simulink model "controller_dev_sg_HIL_noTP"  (R2018b)
settings: configuration reference "Physics" (kept outside this file)
model workspace (MAT data in the model file):
  m = 1000
values from neighbouring files (symbols this model uses):
  bool_activate_Vehicles : value not decoded    [controller_dev_sg.sldd]
  ModObj_ObjList_SendPort = 11004.0    [UDPPortConfig.sldd]
  ModSens_GpsSenDat_SendPort = 3002.0    [UDPPortConfig.sldd]
  sensors_freq_camera = 37.0    [controller_dev_sg.sldd]
  sensors_freq_gps = 20.0    [controller_dev_sg.sldd]
  sensors_freq_imu = 100.0    [controller_dev_sg.sldd]
  sensors_freq_lidar = 12.0    [controller_dev_sg.sldd]
  sensors_freq_radar = 20.0    [controller_dev_sg.sldd]
undefined symbols (not defined in the file or in its folder): activate_VariableFriction, C, tpa_map_Reference, tSPhysics, x0_vehiclepos_start_veh1, x0_vehiclepos_start_veh10, x0_vehiclepos_start_veh2, x0_vehiclepos_start_veh3, x0_vehiclepos_start_veh4, x0_vehiclepos_start_veh5, x0_vehiclepos_start_veh6, x0_vehiclepos_start_veh7, x0_vehiclepos_start_veh8, x0_vehiclepos_start_veh9
libraries: xpcutilitieslib x273, xpcrtudplib x215, aerolibconvert2 x48, simulink x30, etargetslib x26, speedgoatlib_IO612 x7, canmsglib x6, slrtlib x4
(part 3 of 16)

== system controller_dev_sg_HIL_noTP/UDP to Control (Position, IMU, Wheelspeed)4 ==
  VehicleSensorData : Inport
  VehicleSystemStatus : Inport  Port=2
  ActuatorLimitations : Inport  Port=3
  Enable : EnablePort
  Bus Creator : BusCreator  Inputs=14
  Bus Creator2 : BusCreator  Inputs=4
  Bus Selector : BusSelector  OutputSignals=omega_WheelFL_radps,omega_WheelFR_radps,omega_WheelRL_radps,omega_WheelRR_radps,ax_CoGIMU1_mps2,ay_CoGIMU1_mps2,dPsi_YawRateIMU1_radps,Delta_Wheel_rad,p_BrakeF_bar,p_BrakeR_bar,ThrottlePos_perc,T_Engine_Nm,omega_Engine_radps,GearEngaged
  Bus Selector1 : BusSelector  OutputSignals=Hardware,AIDriver,ParkBrakeApplied_b,VehicleReady2Drive
  Bus Selector2 : BusSelector  OutputSignals=SteeringAngleMax_rad,SteeringAngleMin_rad,DriveForceMax_N,DriveForceMin_N
  Byte Packing 1 : xpcutilitieslib/Byte Packing   MaskPackedDataType=uint8  MaskUnpackedDataTypes={'uint16','uint16','uint8','uint8'}  MaskAlignment=1
  Byte Packing 2 : xpcutilitieslib/Byte Packing   MaskPackedDataType=uint8  MaskUnpackedDataTypes={'double'}  MaskAlignment=1
  Byte Packing 3 : xpcutilitieslib/Byte Packing   MaskPackedDataType=uint8  MaskUnpackedDataTypes={'double'}  MaskAlignment=1
  Data Type Conversion{,1..3,8..21} (18 alike) : DataTypeConversion  OutDataTypeStr=double
  Data Type Conversion4 : DataTypeConversion  OutDataTypeStr=uint16
  Data Type Conversion5 : DataTypeConversion  OutDataTypeStr=uint16
  Data Type Conversion6 : DataTypeConversion  OutDataTypeStr=uint8
  Data Type Conversion7 : DataTypeConversion  OutDataTypeStr=uint8
  UDP Send1 : xpcrtudplib/UDP Send  ipAddressVal=10.0.0.20  localPort=40550  toAddress=10.0.0.15  toPort=ModCtrl_VehSenDat_SendPort  sampleTime=-1
      settings: SourceProductName=Simulink Real-Time  SourceProductBaseCode=XP
  UDP Send2 : xpcrtudplib/UDP Send  ipAddressVal=10.0.0.20  localPort=40551  toAddress=10.0.0.15  toPort=ModCtrl_VehSysStat_SendPort  sampleTime=-1
      settings: SourceProductName=Simulink Real-Time  SourceProductBaseCode=XP
  UDP Send3 : xpcrtudplib/UDP Send  ipAddressVal=10.0.0.20  localPort=40552  toAddress=10.0.0.15  toPort=ModCtrl_ActLim_SendPort  sampleTime=-1
      settings: SourceProductName=Simulink Real-Time  SourceProductBaseCode=XP
  Width : Width
  Width1 : Width
  Width2 : Width
  wires:
  VehicleSensorData/1 -> Bus Selector/1
  Byte Packing 3/1 -> UDP Send1/1, Width/1
  Width/1 -> UDP Send1/2
  VehicleSystemStatus/1 -> Bus Selector1/1
  Bus Selector1/1 -> Data Type Conversion4/1  "<Hardware>"
  Bus Selector1/4 -> Data Type Conversion6/1  "<VehicleReady2Drive>"
  Bus Selector1/3 -> Data Type Conversion7/1  "<ParkBrakeApplied_b>"
  Bus Selector1/2 -> Data Type Conversion5/1  "<AIDriver>"
  ActuatorLimitations/1 -> Bus Selector2/1
  Bus Selector2/4 -> Data Type Conversion9/1  "<DriveForceMin_N>"
  Bus Selector2/3 -> Data Type Conversion10/1  "<DriveForceMax_N>"
  Bus Selector2/2 -> Data Type Conversion11/1  "<SteeringAngleMin_rad>"
  Bus Selector2/1 -> Data Type Conversion8/1  "<SteeringAngleMax_rad>"
  Data Type Conversion6/1 -> Byte Packing 1/4
  Data Type Conversion7/1 -> Byte Packing 1/3
  Data Type Conversion5/1 -> Byte Packing 1/2
  Data Type Conversion8/1 -> Bus Creator2/1
  Data Type Conversion11/1 -> Bus Creator2/2
  Data Type Conversion10/1 -> Bus Creator2/3
  Data Type Conversion9/1 -> Bus Creator2/4
  Bus Creator/1 -> Byte Packing 3/1
  Data Type Conversion4/1 -> Byte Packing 1/1
  Bus Creator2/1 -> Byte Packing 2/1
  Byte Packing 1/1 -> UDP Send2/1, Width1/1
  Width1/1 -> UDP Send2/2
  Byte Packing 2/1 -> UDP Send3/1, Width2/1
  Width2/1 -> UDP Send3/2
  Data Type Conversion1/1 -> Bus Creator/4
  Data Type Conversion2/1 -> Bus Creator/3
  Data Type Conversion19/1 -> Bus Creator/12
  Data Type Conversion3/1 -> Bus Creator/2
  Data Type Conversion16/1 -> Bus Creator/11
  Data Type Conversion14/1 -> Bus Creator/5
  Bus Selector/3 -> Data Type Conversion2/1  "<omega_WheelRL_radps>"
  Bus Selector/1 -> Data Type Conversion/1  "<omega_WheelFL_radps>"
  Data Type Conversion13/1 -> Bus Creator/7
  Bus Selector/4 -> Data Type Conversion1/1  "<omega_WheelRR_radps>"
  Bus Selector/2 -> Data Type Conversion3/1  "<omega_WheelFR_radps>"
  Data Type Conversion21/1 -> Bus Creator/9
  Data Type Conversion15/1 -> Bus Creator/8
  Bus Selector/10 -> Data Type Conversion20/1  "<p_BrakeR_bar>"
  Bus Selector/9 -> Data Type Conversion21/1  "<p_BrakeF_bar>"
  Bus Selector/8 -> Data Type Conversion15/1  "<Delta_Wheel_rad>"
  Data Type Conversion12/1 -> Bus Creator/6
  Data Type Conversion17/1 -> Bus Creator/13
  Bus Selector/12 -> Data Type Conversion19/1  "<T_Engine_Nm>"
  Bus Selector/13 -> Data Type Conversion17/1  "<omega_Engine_radps>"
  Bus Selector/11 -> Data Type Conversion16/1  "<ThrottlePos_perc>"
  Bus Selector/7 -> Data Type Conversion13/1  "<dPsi_YawRateIMU1_radps>"
  Data Type Conversion/1 -> Bus Creator/1
  Data Type Conversion20/1 -> Bus Creator/10
  Bus Selector/6 -> Data Type Conversion12/1  "<ay_CoGIMU1_mps2>"
  Data Type Conversion18/1 -> Bus Creator/14
  Bus Selector/5 -> Data Type Conversion14/1  "<ax_CoGIMU1_mps2>"
  Bus Selector/14 -> Data Type Conversion18/1  "<GearEngaged>"

== system controller_dev_sg_HIL_noTP/UDP to Control (Position, IMU, Wheelspeed)5 ==
  VehicleSensorData : Inport
  VehicleSystemStatus : Inport  Port=2
  ActuatorLimitations : Inport  Port=3
  Enable : EnablePort
  Bus Creator : BusCreator  Inputs=14
  Bus Creator2 : BusCreator  Inputs=4
  Bus Selector : BusSelector  OutputSignals=omega_WheelFL_radps,omega_WheelFR_radps,omega_WheelRL_radps,omega_WheelRR_radps,ax_CoGIMU1_mps2,ay_CoGIMU1_mps2,dPsi_YawRateIMU1_radps,Delta_Wheel_rad,p_BrakeF_bar,p_BrakeR_bar,ThrottlePos_perc,T_Engine_Nm,omega_Engine_radps,GearEngaged
  Bus Selector1 : BusSelector  OutputSignals=Hardware,AIDriver,ParkBrakeApplied_b,VehicleReady2Drive
  Bus Selector2 : BusSelector  OutputSignals=SteeringAngleMax_rad,SteeringAngleMin_rad,DriveForceMax_N,DriveForceMin_N
  Byte Packing 1 : xpcutilitieslib/Byte Packing   MaskPackedDataType=uint8  MaskUnpackedDataTypes={'uint16','uint16','uint8','uint8'}  MaskAlignment=1
  Byte Packing 2 : xpcutilitieslib/Byte Packing   MaskPackedDataType=uint8  MaskUnpackedDataTypes={'double'}  MaskAlignment=1
  Byte Packing 3 : xpcutilitieslib/Byte Packing   MaskPackedDataType=uint8  MaskUnpackedDataTypes={'double'}  MaskAlignment=1
  Data Type Conversion{,1..3,8..21} (18 alike) : DataTypeConversion  OutDataTypeStr=double
  Data Type Conversion4 : DataTypeConversion  OutDataTypeStr=uint16
  Data Type Conversion5 : DataTypeConversion  OutDataTypeStr=uint16
  Data Type Conversion6 : DataTypeConversion  OutDataTypeStr=uint8
  Data Type Conversion7 : DataTypeConversion  OutDataTypeStr=uint8
  UDP Send1 : xpcrtudplib/UDP Send  ipAddressVal=10.0.0.20  localPort=40560  toAddress=10.0.0.16  toPort=ModCtrl_VehSenDat_SendPort  sampleTime=-1
      settings: SourceProductName=Simulink Real-Time  SourceProductBaseCode=XP
  UDP Send2 : xpcrtudplib/UDP Send  ipAddressVal=10.0.0.20  localPort=40561  toAddress=10.0.0.16  toPort=ModCtrl_VehSysStat_SendPort  sampleTime=-1
      settings: SourceProductName=Simulink Real-Time  SourceProductBaseCode=XP
  UDP Send3 : xpcrtudplib/UDP Send  ipAddressVal=10.0.0.20  localPort=40562  toAddress=10.0.0.16  toPort=ModCtrl_ActLim_SendPort  sampleTime=-1
      settings: SourceProductName=Simulink Real-Time  SourceProductBaseCode=XP
  Width : Width
  Width1 : Width
  Width2 : Width
  wires:
  VehicleSensorData/1 -> Bus Selector/1
  Byte Packing 3/1 -> UDP Send1/1, Width/1
  Width/1 -> UDP Send1/2
  VehicleSystemStatus/1 -> Bus Selector1/1
  Bus Selector1/1 -> Data Type Conversion4/1  "<Hardware>"
  Bus Selector1/4 -> Data Type Conversion6/1  "<VehicleReady2Drive>"
  Bus Selector1/3 -> Data Type Conversion7/1  "<ParkBrakeApplied_b>"
  Bus Selector1/2 -> Data Type Conversion5/1  "<AIDriver>"
  ActuatorLimitations/1 -> Bus Selector2/1
  Bus Selector2/4 -> Data Type Conversion9/1  "<DriveForceMin_N>"
  Bus Selector2/3 -> Data Type Conversion10/1  "<DriveForceMax_N>"
  Bus Selector2/2 -> Data Type Conversion11/1  "<SteeringAngleMin_rad>"
  Bus Selector2/1 -> Data Type Conversion8/1  "<SteeringAngleMax_rad>"
  Data Type Conversion6/1 -> Byte Packing 1/4
  Data Type Conversion7/1 -> Byte Packing 1/3
  Data Type Conversion5/1 -> Byte Packing 1/2
  Data Type Conversion8/1 -> Bus Creator2/1
  Data Type Conversion11/1 -> Bus Creator2/2
  Data Type Conversion10/1 -> Bus Creator2/3
  Data Type Conversion9/1 -> Bus Creator2/4
  Bus Creator/1 -> Byte Packing 3/1
  Data Type Conversion4/1 -> Byte Packing 1/1
  Bus Creator2/1 -> Byte Packing 2/1
  Byte Packing 1/1 -> UDP Send2/1, Width1/1
  Width1/1 -> UDP Send2/2
  Byte Packing 2/1 -> UDP Send3/1, Width2/1
  Width2/1 -> UDP Send3/2
  Data Type Conversion1/1 -> Bus Creator/4
  Data Type Conversion2/1 -> Bus Creator/3
  Data Type Conversion19/1 -> Bus Creator/12
  Data Type Conversion3/1 -> Bus Creator/2
  Data Type Conversion16/1 -> Bus Creator/11
  Data Type Conversion14/1 -> Bus Creator/5
  Bus Selector/3 -> Data Type Conversion2/1  "<omega_WheelRL_radps>"
  Bus Selector/1 -> Data Type Conversion/1  "<omega_WheelFL_radps>"
  Data Type Conversion13/1 -> Bus Creator/7
  Bus Selector/4 -> Data Type Conversion1/1  "<omega_WheelRR_radps>"
  Bus Selector/2 -> Data Type Conversion3/1  "<omega_WheelFR_radps>"
  Data Type Conversion21/1 -> Bus Creator/9
  Data Type Conversion15/1 -> Bus Creator/8
  Bus Selector/10 -> Data Type Conversion20/1  "<p_BrakeR_bar>"
  Bus Selector/9 -> Data Type Conversion21/1  "<p_BrakeF_bar>"
  Bus Selector/8 -> Data Type Conversion15/1  "<Delta_Wheel_rad>"
  Data Type Conversion12/1 -> Bus Creator/6
  Data Type Conversion17/1 -> Bus Creator/13
  Bus Selector/12 -> Data Type Conversion19/1  "<T_Engine_Nm>"
  Bus Selector/13 -> Data Type Conversion17/1  "<omega_Engine_radps>"
  Bus Selector/11 -> Data Type Conversion16/1  "<ThrottlePos_perc>"
  Bus Selector/7 -> Data Type Conversion13/1  "<dPsi_YawRateIMU1_radps>"
  Data Type Conversion/1 -> Bus Creator/1
  Data Type Conversion20/1 -> Bus Creator/10
  Bus Selector/6 -> Data Type Conversion12/1  "<ay_CoGIMU1_mps2>"
  Data Type Conversion18/1 -> Bus Creator/14
  Bus Selector/5 -> Data Type Conversion14/1  "<ax_CoGIMU1_mps2>"
  Bus Selector/14 -> Data Type Conversion18/1  "<GearEngaged>"

== system controller_dev_sg_HIL_noTP/UDP to Control (Position, IMU, Wheelspeed)6 ==
  VehicleSensorData : Inport
  VehicleSystemStatus : Inport  Port=2
  ActuatorLimitations : Inport  Port=3
  Enable : EnablePort
  Bus Creator : BusCreator  Inputs=14
  Bus Creator2 : BusCreator  Inputs=4
  Bus Selector : BusSelector  OutputSignals=omega_WheelFL_radps,omega_WheelFR_radps,omega_WheelRL_radps,omega_WheelRR_radps,ax_CoGIMU1_mps2,ay_CoGIMU1_mps2,dPsi_YawRateIMU1_radps,Delta_Wheel_rad,p_BrakeF_bar,p_BrakeR_bar,ThrottlePos_perc,T_Engine_Nm,omega_Engine_radps,GearEngaged
  Bus Selector1 : BusSelector  OutputSignals=Hardware,AIDriver,ParkBrakeApplied_b,VehicleReady2Drive
  Bus Selector2 : BusSelector  OutputSignals=SteeringAngleMax_rad,SteeringAngleMin_rad,DriveForceMax_N,DriveForceMin_N
  Byte Packing 1 : xpcutilitieslib/Byte Packing   MaskPackedDataType=uint8  MaskUnpackedDataTypes={'uint16','uint16','uint8','uint8'}  MaskAlignment=1
  Byte Packing 2 : xpcutilitieslib/Byte Packing   MaskPackedDataType=uint8  MaskUnpackedDataTypes={'double'}  MaskAlignment=1
  Byte Packing 3 : xpcutilitieslib/Byte Packing   MaskPackedDataType=uint8  MaskUnpackedDataTypes={'double'}  MaskAlignment=1
  Data Type Conversion{,1..3,8..21} (18 alike) : DataTypeConversion  OutDataTypeStr=double
  Data Type Conversion4 : DataTypeConversion  OutDataTypeStr=uint16
  Data Type Conversion5 : DataTypeConversion  OutDataTypeStr=uint16
  Data Type Conversion6 : DataTypeConversion  OutDataTypeStr=uint8
  Data Type Conversion7 : DataTypeConversion  OutDataTypeStr=uint8
  UDP Send1 : xpcrtudplib/UDP Send  ipAddressVal=10.0.0.20  localPort=40570  toAddress=10.0.0.17  toPort=ModCtrl_VehSenDat_SendPort  sampleTime=-1
      settings: SourceProductName=Simulink Real-Time  SourceProductBaseCode=XP
  UDP Send2 : xpcrtudplib/UDP Send  ipAddressVal=10.0.0.20  localPort=40571  toAddress=10.0.0.17  toPort=ModCtrl_VehSysStat_SendPort  sampleTime=-1
      settings: SourceProductName=Simulink Real-Time  SourceProductBaseCode=XP
  UDP Send3 : xpcrtudplib/UDP Send  ipAddressVal=10.0.0.20  localPort=40572  toAddress=10.0.0.17  toPort=ModCtrl_ActLim_SendPort  sampleTime=-1
      settings: SourceProductName=Simulink Real-Time  SourceProductBaseCode=XP
  Width : Width
  Width1 : Width
  Width2 : Width
  wires:
  VehicleSensorData/1 -> Bus Selector/1
  Byte Packing 3/1 -> UDP Send1/1, Width/1
  Width/1 -> UDP Send1/2
  VehicleSystemStatus/1 -> Bus Selector1/1
  Bus Selector1/1 -> Data Type Conversion4/1  "<Hardware>"
  Bus Selector1/4 -> Data Type Conversion6/1  "<VehicleReady2Drive>"
  Bus Selector1/3 -> Data Type Conversion7/1  "<ParkBrakeApplied_b>"
  Bus Selector1/2 -> Data Type Conversion5/1  "<AIDriver>"
  ActuatorLimitations/1 -> Bus Selector2/1
  Bus Selector2/4 -> Data Type Conversion9/1  "<DriveForceMin_N>"
  Bus Selector2/3 -> Data Type Conversion10/1  "<DriveForceMax_N>"
  Bus Selector2/2 -> Data Type Conversion11/1  "<SteeringAngleMin_rad>"
  Bus Selector2/1 -> Data Type Conversion8/1  "<SteeringAngleMax_rad>"
  Data Type Conversion6/1 -> Byte Packing 1/4
  Data Type Conversion7/1 -> Byte Packing 1/3
  Data Type Conversion5/1 -> Byte Packing 1/2
  Data Type Conversion8/1 -> Bus Creator2/1
  Data Type Conversion11/1 -> Bus Creator2/2
  Data Type Conversion10/1 -> Bus Creator2/3
  Data Type Conversion9/1 -> Bus Creator2/4
  Bus Creator/1 -> Byte Packing 3/1
  Data Type Conversion4/1 -> Byte Packing 1/1
  Bus Creator2/1 -> Byte Packing 2/1
  Byte Packing 1/1 -> UDP Send2/1, Width1/1
  Width1/1 -> UDP Send2/2
  Byte Packing 2/1 -> UDP Send3/1, Width2/1
  Width2/1 -> UDP Send3/2
  Data Type Conversion1/1 -> Bus Creator/4
  Data Type Conversion2/1 -> Bus Creator/3
  Data Type Conversion19/1 -> Bus Creator/12
  Data Type Conversion3/1 -> Bus Creator/2
  Data Type Conversion16/1 -> Bus Creator/11
  Data Type Conversion14/1 -> Bus Creator/5
  Bus Selector/3 -> Data Type Conversion2/1  "<omega_WheelRL_radps>"
  Bus Selector/1 -> Data Type Conversion/1  "<omega_WheelFL_radps>"
  Data Type Conversion13/1 -> Bus Creator/7
  Bus Selector/4 -> Data Type Conversion1/1  "<omega_WheelRR_radps>"
  Bus Selector/2 -> Data Type Conversion3/1  "<omega_WheelFR_radps>"
  Data Type Conversion21/1 -> Bus Creator/9
  Data Type Conversion15/1 -> Bus Creator/8
  Bus Selector/10 -> Data Type Conversion20/1  "<p_BrakeR_bar>"
  Bus Selector/9 -> Data Type Conversion21/1  "<p_BrakeF_bar>"
  Bus Selector/8 -> Data Type Conversion15/1  "<Delta_Wheel_rad>"
  Data Type Conversion12/1 -> Bus Creator/6
  Data Type Conversion17/1 -> Bus Creator/13
  Bus Selector/12 -> Data Type Conversion19/1  "<T_Engine_Nm>"
  Bus Selector/13 -> Data Type Conversion17/1  "<omega_Engine_radps>"
  Bus Selector/11 -> Data Type Conversion16/1  "<ThrottlePos_perc>"
  Bus Selector/7 -> Data Type Conversion13/1  "<dPsi_YawRateIMU1_radps>"
  Data Type Conversion/1 -> Bus Creator/1
  Data Type Conversion20/1 -> Bus Creator/10
  Bus Selector/6 -> Data Type Conversion12/1  "<ay_CoGIMU1_mps2>"
  Data Type Conversion18/1 -> Bus Creator/14
  Bus Selector/5 -> Data Type Conversion14/1  "<ax_CoGIMU1_mps2>"
  Bus Selector/14 -> Data Type Conversion18/1  "<GearEngaged>"

== system controller_dev_sg_HIL_noTP/UDP to Control (Position, IMU, Wheelspeed)7 ==
  VehicleSensorData : Inport
  VehicleSystemStatus : Inport  Port=2
  ActuatorLimitations : Inport  Port=3
  Enable : EnablePort
  Bus Creator : BusCreator  Inputs=14
  Bus Creator2 : BusCreator  Inputs=4
  Bus Selector : BusSelector  OutputSignals=omega_WheelFL_radps,omega_WheelFR_radps,omega_WheelRL_radps,omega_WheelRR_radps,ax_CoGIMU1_mps2,ay_CoGIMU1_mps2,dPsi_YawRateIMU1_radps,Delta_Wheel_rad,p_BrakeF_bar,p_BrakeR_bar,ThrottlePos_perc,T_Engine_Nm,omega_Engine_radps,GearEngaged
  Bus Selector1 : BusSelector  OutputSignals=Hardware,AIDriver,ParkBrakeApplied_b,VehicleReady2Drive
  Bus Selector2 : BusSelector  OutputSignals=SteeringAngleMax_rad,SteeringAngleMin_rad,DriveForceMax_N,DriveForceMin_N
  Byte Packing 1 : xpcutilitieslib/Byte Packing   MaskPackedDataType=uint8  MaskUnpackedDataTypes={'uint16','uint16','uint8','uint8'}  MaskAlignment=1
  Byte Packing 2 : xpcutilitieslib/Byte Packing   MaskPackedDataType=uint8  MaskUnpackedDataTypes={'double'}  MaskAlignment=1
  Byte Packing 3 : xpcutilitieslib/Byte Packing   MaskPackedDataType=uint8  MaskUnpackedDataTypes={'double'}  MaskAlignment=1
  Data Type Conversion{,1..3,8..21} (18 alike) : DataTypeConversion  OutDataTypeStr=double
  Data Type Conversion4 : DataTypeConversion  OutDataTypeStr=uint16
  Data Type Conversion5 : DataTypeConversion  OutDataTypeStr=uint16
  Data Type Conversion6 : DataTypeConversion  OutDataTypeStr=uint8
  Data Type Conversion7 : DataTypeConversion  OutDataTypeStr=uint8
  UDP Send1 : xpcrtudplib/UDP Send  ipAddressVal=10.0.0.20  localPort=40580  toAddress=10.0.0.18  toPort=ModCtrl_VehSenDat_SendPort  sampleTime=-1
      settings: SourceProductName=Simulink Real-Time  SourceProductBaseCode=XP
  UDP Send2 : xpcrtudplib/UDP Send  ipAddressVal=10.0.0.20  localPort=40581  toAddress=10.0.0.18  toPort=ModCtrl_VehSysStat_SendPort  sampleTime=-1
      settings: SourceProductName=Simulink Real-Time  SourceProductBaseCode=XP
  UDP Send3 : xpcrtudplib/UDP Send  ipAddressVal=10.0.0.20  localPort=40582  toAddress=10.0.0.18  toPort=ModCtrl_ActLim_SendPort  sampleTime=-1
      settings: SourceProductName=Simulink Real-Time  SourceProductBaseCode=XP
  Width : Width
  Width1 : Width
  Width2 : Width
  wires:
  VehicleSensorData/1 -> Bus Selector/1
  Byte Packing 3/1 -> UDP Send1/1, Width/1
  Width/1 -> UDP Send1/2
  VehicleSystemStatus/1 -> Bus Selector1/1
  Bus Selector1/1 -> Data Type Conversion4/1  "<Hardware>"
  Bus Selector1/4 -> Data Type Conversion6/1  "<VehicleReady2Drive>"
  Bus Selector1/3 -> Data Type Conversion7/1  "<ParkBrakeApplied_b>"
  Bus Selector1/2 -> Data Type Conversion5/1  "<AIDriver>"
  ActuatorLimitations/1 -> Bus Selector2/1
  Bus Selector2/4 -> Data Type Conversion9/1  "<DriveForceMin_N>"
  Bus Selector2/3 -> Data Type Conversion10/1  "<DriveForceMax_N>"
  Bus Selector2/2 -> Data Type Conversion11/1  "<SteeringAngleMin_rad>"
  Bus Selector2/1 -> Data Type Conversion8/1  "<SteeringAngleMax_rad>"
  Data Type Conversion6/1 -> Byte Packing 1/4
  Data Type Conversion7/1 -> Byte Packing 1/3
  Data Type Conversion5/1 -> Byte Packing 1/2
  Data Type Conversion8/1 -> Bus Creator2/1
  Data Type Conversion11/1 -> Bus Creator2/2
  Data Type Conversion10/1 -> Bus Creator2/3
  Data Type Conversion9/1 -> Bus Creator2/4
  Bus Creator/1 -> Byte Packing 3/1
  Data Type Conversion4/1 -> Byte Packing 1/1
  Bus Creator2/1 -> Byte Packing 2/1
  Byte Packing 1/1 -> UDP Send2/1, Width1/1
  Width1/1 -> UDP Send2/2
  Byte Packing 2/1 -> UDP Send3/1, Width2/1
  Width2/1 -> UDP Send3/2
  Data Type Conversion1/1 -> Bus Creator/4
  Data Type Conversion2/1 -> Bus Creator/3
  Data Type Conversion19/1 -> Bus Creator/12
  Data Type Conversion3/1 -> Bus Creator/2
  Data Type Conversion16/1 -> Bus Creator/11
  Data Type Conversion14/1 -> Bus Creator/5
  Bus Selector/3 -> Data Type Conversion2/1  "<omega_WheelRL_radps>"
  Bus Selector/1 -> Data Type Conversion/1  "<omega_WheelFL_radps>"
  Data Type Conversion13/1 -> Bus Creator/7
  Bus Selector/4 -> Data Type Conversion1/1  "<omega_WheelRR_radps>"
  Bus Selector/2 -> Data Type Conversion3/1  "<omega_WheelFR_radps>"
  Data Type Conversion21/1 -> Bus Creator/9
  Data Type Conversion15/1 -> Bus Creator/8
  Bus Selector/10 -> Data Type Conversion20/1  "<p_BrakeR_bar>"
  Bus Selector/9 -> Data Type Conversion21/1  "<p_BrakeF_bar>"
  Bus Selector/8 -> Data Type Conversion15/1  "<Delta_Wheel_rad>"
  Data Type Conversion12/1 -> Bus Creator/6
  Data Type Conversion17/1 -> Bus Creator/13
  Bus Selector/12 -> Data Type Conversion19/1  "<T_Engine_Nm>"
  Bus Selector/13 -> Data Type Conversion17/1  "<omega_Engine_radps>"
  Bus Selector/11 -> Data Type Conversion16/1  "<ThrottlePos_perc>"
  Bus Selector/7 -> Data Type Conversion13/1  "<dPsi_YawRateIMU1_radps>"
  Data Type Conversion/1 -> Bus Creator/1
  Data Type Conversion20/1 -> Bus Creator/10
  Bus Selector/6 -> Data Type Conversion12/1  "<ay_CoGIMU1_mps2>"
  Data Type Conversion18/1 -> Bus Creator/14
  Bus Selector/5 -> Data Type Conversion14/1  "<ax_CoGIMU1_mps2>"
  Bus Selector/14 -> Data Type Conversion18/1  "<GearEngaged>"

== system controller_dev_sg_HIL_noTP/UDP to Mapping and Localization (Position, IMU, Wheelspeed) ==
  VehicleSensorData : Inport
  Enable : EnablePort
  Bus Creator : BusCreator  Inputs=12
  Bus Selector : BusSelector  OutputSignals=x_Loc1_m,y_Loc1_m,psi_YawAngleLoc1_rad,vx_CoGVel1_mps,vy_CoGVel1_mps,dPsi_YawRateIMU1_radps,ax_CoGIMU1_mps2,ay_CoGIMU1_mps2,omega_WheelFL_radps,omega_WheelFR_radps,omega_WheelRL_radps,omega_WheelRR_radps
  Byte Packing 3 : xpcutilitieslib/Byte Packing   MaskPackedDataType=uint8  MaskUnpackedDataTypes={'double'}  MaskAlignment=1
  Data Type Conversion{,1..8,12..14} (12 alike) : DataTypeConversion  OutDataTypeStr=double
  UDP Send1 : xpcrtudplib/UDP Send  ipAddressVal=10.0.0.20  localPort=40513  toAddress=10.0.0.11  toPort=ModMapLoc_VehSenDat_SendPort  sampleTime=-1
      settings: SourceProductName=Simulink Real-Time  SourceProductBaseCode=XP
  Width : Width
  wires:
  VehicleSensorData/1 -> Bus Selector/1
  Byte Packing 3/1 -> Width/1, UDP Send1/1
  Width/1 -> UDP Send1/2
  Bus Creator/1 -> Byte Packing 3/1
  Bus Selector/12 -> Data Type Conversion13/1  "<omega_WheelRR_radps>"
  Bus Selector/11 -> Data Type Conversion12/1  "<omega_WheelRL_radps>"
  Bus Selector/10 -> Data Type Conversion14/1  "<omega_WheelFR_radps>"
  Bus Selector/9 -> Data Type Conversion1/1  "<omega_WheelFL_radps>"
  Bus Selector/7 -> Data Type Conversion3/1  "<ax_CoGIMU1_mps2>"
  Bus Selector/8 -> Data Type Conversion2/1  "<ay_CoGIMU1_mps2>"
  Bus Selector/6 -> Data Type Conversion/1  "<dPsi_YawRateIMU1_radps>"
  Bus Selector/1 -> Data Type Conversion4/1  "<x_Loc1_m>"
  Bus Selector/2 -> Data Type Conversion8/1  "<y_Loc1_m>"
  Bus Selector/3 -> Data Type Conversion7/1  "<psi_YawAngleLoc1_rad>"
  Bus Selector/4 -> Data Type Conversion5/1  "<vx_CoGVel1_mps>"
  Bus Selector/5 -> Data Type Conversion6/1  "<vy_CoGVel1_mps>"
  Data Type Conversion12/1 -> Bus Creator/11
  Data Type Conversion13/1 -> Bus Creator/12
  Data Type Conversion14/1 -> Bus Creator/10
  Data Type Conversion1/1 -> Bus Creator/9
  Data Type Conversion3/1 -> Bus Creator/7
  Data Type Conversion2/1 -> Bus Creator/8
  Data Type Conversion/1 -> Bus Creator/6
  Data Type Conversion6/1 -> Bus Creator/5
  Data Type Conversion5/1 -> Bus Creator/4
  Data Type Conversion7/1 -> Bus Creator/3
  Data Type Conversion8/1 -> Bus Creator/2
  Data Type Conversion4/1 -> Bus Creator/1

== system controller_dev_sg_HIL_noTP/UDP to Mapping and Localization (Position, IMU, Wheelspeed)1 ==
  VehicleSensorData : Inport
  Enable : EnablePort
  Bus Creator : BusCreator  Inputs=12
  Bus Selector : BusSelector  OutputSignals=x_Loc1_m,y_Loc1_m,psi_YawAngleLoc1_rad,vx_CoGVel1_mps,vy_CoGVel1_mps,dPsi_YawRateIMU1_radps,ax_CoGIMU1_mps2,ay_CoGIMU1_mps2,omega_WheelFL_radps,omega_WheelFR_radps,omega_WheelRL_radps,omega_WheelRR_radps
  Byte Packing 3 : xpcutilitieslib/Byte Packing   MaskPackedDataType=uint8  MaskUnpackedDataTypes={'double'}  MaskAlignment=1
  Data Type Conversion{,1..8,12..14} (12 alike) : DataTypeConversion  OutDataTypeStr=double
  UDP Send1 : xpcrtudplib/UDP Send  ipAddressVal=10.0.0.20  localPort=40523  toAddress=10.0.0.12  toPort=ModMapLoc_VehSenDat_SendPort  sampleTime=-1
      settings: SourceProductName=Simulink Real-Time  SourceProductBaseCode=XP
  Width : Width
  wires:
  VehicleSensorData/1 -> Bus Selector/1
  Byte Packing 3/1 -> Width/1, UDP Send1/1
  Width/1 -> UDP Send1/2
  Bus Creator/1 -> Byte Packing 3/1
  Bus Selector/12 -> Data Type Conversion13/1  "<omega_WheelRR_radps>"
  Bus Selector/11 -> Data Type Conversion12/1  "<omega_WheelRL_radps>"
  Bus Selector/10 -> Data Type Conversion14/1  "<omega_WheelFR_radps>"
  Bus Selector/9 -> Data Type Conversion1/1  "<omega_WheelFL_radps>"
  Bus Selector/7 -> Data Type Conversion3/1  "<ax_CoGIMU1_mps2>"
  Bus Selector/8 -> Data Type Conversion2/1  "<ay_CoGIMU1_mps2>"
  Bus Selector/6 -> Data Type Conversion/1  "<dPsi_YawRateIMU1_radps>"
  Bus Selector/1 -> Data Type Conversion4/1  "<x_Loc1_m>"
  Bus Selector/2 -> Data Type Conversion8/1  "<y_Loc1_m>"
  Bus Selector/3 -> Data Type Conversion7/1  "<psi_YawAngleLoc1_rad>"
  Bus Selector/4 -> Data Type Conversion5/1  "<vx_CoGVel1_mps>"
  Bus Selector/5 -> Data Type Conversion6/1  "<vy_CoGVel1_mps>"
  Data Type Conversion12/1 -> Bus Creator/11
  Data Type Conversion13/1 -> Bus Creator/12
  Data Type Conversion14/1 -> Bus Creator/10
  Data Type Conversion1/1 -> Bus Creator/9
  Data Type Conversion3/1 -> Bus Creator/7
  Data Type Conversion2/1 -> Bus Creator/8
  Data Type Conversion/1 -> Bus Creator/6
  Data Type Conversion6/1 -> Bus Creator/5
  Data Type Conversion5/1 -> Bus Creator/4
  Data Type Conversion7/1 -> Bus Creator/3
  Data Type Conversion8/1 -> Bus Creator/2
  Data Type Conversion4/1 -> Bus Creator/1

== system controller_dev_sg_HIL_noTP/UDP to Mapping and Localization (Position, IMU, Wheelspeed)2 ==
  VehicleSensorData : Inport
  Enable : EnablePort
  Bus Creator : BusCreator  Inputs=12
  Bus Selector : BusSelector  OutputSignals=x_Loc1_m,y_Loc1_m,psi_YawAngleLoc1_rad,vx_CoGVel1_mps,vy_CoGVel1_mps,dPsi_YawRateIMU1_radps,ax_CoGIMU1_mps2,ay_CoGIMU1_mps2,omega_WheelFL_radps,omega_WheelFR_radps,omega_WheelRL_radps,omega_WheelRR_radps
  Byte Packing 3 : xpcutilitieslib/Byte Packing   MaskPackedDataType=uint8  MaskUnpackedDataTypes={'double'}  MaskAlignment=1
  Data Type Conversion{,1..8,12..14} (12 alike) : DataTypeConversion  OutDataTypeStr=double
  UDP Send1 : xpcrtudplib/UDP Send  ipAddressVal=10.0.0.20  localPort=40533  toAddress=10.0.0.13  toPort=ModMapLoc_VehSenDat_SendPort  sampleTime=-1
      settings: SourceProductName=Simulink Real-Time  SourceProductBaseCode=XP
  Width : Width
  wires:
  VehicleSensorData/1 -> Bus Selector/1
  Byte Packing 3/1 -> Width/1, UDP Send1/1
  Width/1 -> UDP Send1/2
  Bus Creator/1 -> Byte Packing 3/1
  Bus Selector/12 -> Data Type Conversion13/1  "<omega_WheelRR_radps>"
  Bus Selector/11 -> Data Type Conversion12/1  "<omega_WheelRL_radps>"
  Bus Selector/10 -> Data Type Conversion14/1  "<omega_WheelFR_radps>"
  Bus Selector/9 -> Data Type Conversion1/1  "<omega_WheelFL_radps>"
  Bus Selector/7 -> Data Type Conversion3/1  "<ax_CoGIMU1_mps2>"
  Bus Selector/8 -> Data Type Conversion2/1  "<ay_CoGIMU1_mps2>"
  Bus Selector/6 -> Data Type Conversion/1  "<dPsi_YawRateIMU1_radps>"
  Bus Selector/1 -> Data Type Conversion4/1  "<x_Loc1_m>"
  Bus Selector/2 -> Data Type Conversion8/1  "<y_Loc1_m>"
  Bus Selector/3 -> Data Type Conversion7/1  "<psi_YawAngleLoc1_rad>"
  Bus Selector/4 -> Data Type Conversion5/1  "<vx_CoGVel1_mps>"
  Bus Selector/5 -> Data Type Conversion6/1  "<vy_CoGVel1_mps>"
  Data Type Conversion12/1 -> Bus Creator/11
  Data Type Conversion13/1 -> Bus Creator/12
  Data Type Conversion14/1 -> Bus Creator/10
  Data Type Conversion1/1 -> Bus Creator/9
  Data Type Conversion3/1 -> Bus Creator/7
  Data Type Conversion2/1 -> Bus Creator/8
  Data Type Conversion/1 -> Bus Creator/6
  Data Type Conversion6/1 -> Bus Creator/5
  Data Type Conversion5/1 -> Bus Creator/4
  Data Type Conversion7/1 -> Bus Creator/3
  Data Type Conversion8/1 -> Bus Creator/2
  Data Type Conversion4/1 -> Bus Creator/1

== system controller_dev_sg_HIL_noTP/UDP to Mapping and Localization (Position, IMU, Wheelspeed)3 ==
  VehicleSensorData : Inport
  Enable : EnablePort
  Bus Creator : BusCreator  Inputs=12
  Bus Selector : BusSelector  OutputSignals=x_Loc1_m,y_Loc1_m,psi_YawAngleLoc1_rad,vx_CoGVel1_mps,vy_CoGVel1_mps,dPsi_YawRateIMU1_radps,ax_CoGIMU1_mps2,ay_CoGIMU1_mps2,omega_WheelFL_radps,omega_WheelFR_radps,omega_WheelRL_radps,omega_WheelRR_radps
  Byte Packing 3 : xpcutilitieslib/Byte Packing   MaskPackedDataType=uint8  MaskUnpackedDataTypes={'double'}  MaskAlignment=1
  Data Type Conversion{,1..8,12..14} (12 alike) : DataTypeConversion  OutDataTypeStr=double
  UDP Send1 : xpcrtudplib/UDP Send  ipAddressVal=10.0.0.20  localPort=40543  toAddress=10.0.0.14  toPort=ModMapLoc_VehSenDat_SendPort  sampleTime=-1
      settings: SourceProductName=Simulink Real-Time  SourceProductBaseCode=XP
  Width : Width
  wires:
  VehicleSensorData/1 -> Bus Selector/1
  Byte Packing 3/1 -> Width/1, UDP Send1/1
  Width/1 -> UDP Send1/2
  Bus Creator/1 -> Byte Packing 3/1
  Bus Selector/12 -> Data Type Conversion13/1  "<omega_WheelRR_radps>"
  Bus Selector/11 -> Data Type Conversion12/1  "<omega_WheelRL_radps>"
  Bus Selector/10 -> Data Type Conversion14/1  "<omega_WheelFR_radps>"
  Bus Selector/9 -> Data Type Conversion1/1  "<omega_WheelFL_radps>"
  Bus Selector/7 -> Data Type Conversion3/1  "<ax_CoGIMU1_mps2>"
  Bus Selector/8 -> Data Type Conversion2/1  "<ay_CoGIMU1_mps2>"
  Bus Selector/6 -> Data Type Conversion/1  "<dPsi_YawRateIMU1_radps>"
  Bus Selector/1 -> Data Type Conversion4/1  "<x_Loc1_m>"
  Bus Selector/2 -> Data Type Conversion8/1  "<y_Loc1_m>"
  Bus Selector/3 -> Data Type Conversion7/1  "<psi_YawAngleLoc1_rad>"
  Bus Selector/4 -> Data Type Conversion5/1  "<vx_CoGVel1_mps>"
  Bus Selector/5 -> Data Type Conversion6/1  "<vy_CoGVel1_mps>"
  Data Type Conversion12/1 -> Bus Creator/11
  Data Type Conversion13/1 -> Bus Creator/12
  Data Type Conversion14/1 -> Bus Creator/10
  Data Type Conversion1/1 -> Bus Creator/9
  Data Type Conversion3/1 -> Bus Creator/7
  Data Type Conversion2/1 -> Bus Creator/8
  Data Type Conversion/1 -> Bus Creator/6
  Data Type Conversion6/1 -> Bus Creator/5
  Data Type Conversion5/1 -> Bus Creator/4
  Data Type Conversion7/1 -> Bus Creator/3
  Data Type Conversion8/1 -> Bus Creator/2
  Data Type Conversion4/1 -> Bus Creator/1

== system controller_dev_sg_HIL_noTP/UDP to Mapping and Localization (Position, IMU, Wheelspeed)4 ==
  VehicleSensorData : Inport
  Enable : EnablePort
  Bus Creator : BusCreator  Inputs=12
  Bus Selector : BusSelector  OutputSignals=x_Loc1_m,y_Loc1_m,psi_YawAngleLoc1_rad,vx_CoGVel1_mps,vy_CoGVel1_mps,dPsi_YawRateIMU1_radps,ax_CoGIMU1_mps2,ay_CoGIMU1_mps2,omega_WheelFL_radps,omega_WheelFR_radps,omega_WheelRL_radps,omega_WheelRR_radps
  Byte Packing 3 : xpcutilitieslib/Byte Packing   MaskPackedDataType=uint8  MaskUnpackedDataTypes={'double'}  MaskAlignment=1
  Data Type Conversion{,1..8,12..14} (12 alike) : DataTypeConversion  OutDataTypeStr=double
  UDP Send1 : xpcrtudplib/UDP Send  ipAddressVal=10.0.0.20  localPort=40553  toAddress=10.0.0.15  toPort=ModMapLoc_VehSenDat_SendPort  sampleTime=-1
      settings: SourceProductName=Simulink Real-Time  SourceProductBaseCode=XP
  Width : Width
  wires:
  VehicleSensorData/1 -> Bus Selector/1
  Byte Packing 3/1 -> Width/1, UDP Send1/1
  Width/1 -> UDP Send1/2
  Bus Creator/1 -> Byte Packing 3/1
  Bus Selector/12 -> Data Type Conversion13/1  "<omega_WheelRR_radps>"
  Bus Selector/11 -> Data Type Conversion12/1  "<omega_WheelRL_radps>"
  Bus Selector/10 -> Data Type Conversion14/1  "<omega_WheelFR_radps>"
  Bus Selector/9 -> Data Type Conversion1/1  "<omega_WheelFL_radps>"
  Bus Selector/7 -> Data Type Conversion3/1  "<ax_CoGIMU1_mps2>"
  Bus Selector/8 -> Data Type Conversion2/1  "<ay_CoGIMU1_mps2>"
  Bus Selector/6 -> Data Type Conversion/1  "<dPsi_YawRateIMU1_radps>"
  Bus Selector/1 -> Data Type Conversion4/1  "<x_Loc1_m>"
  Bus Selector/2 -> Data Type Conversion8/1  "<y_Loc1_m>"
  Bus Selector/3 -> Data Type Conversion7/1  "<psi_YawAngleLoc1_rad>"
  Bus Selector/4 -> Data Type Conversion5/1  "<vx_CoGVel1_mps>"
  Bus Selector/5 -> Data Type Conversion6/1  "<vy_CoGVel1_mps>"
  Data Type Conversion12/1 -> Bus Creator/11
  Data Type Conversion13/1 -> Bus Creator/12
  Data Type Conversion14/1 -> Bus Creator/10
  Data Type Conversion1/1 -> Bus Creator/9
  Data Type Conversion3/1 -> Bus Creator/7
  Data Type Conversion2/1 -> Bus Creator/8
  Data Type Conversion/1 -> Bus Creator/6
  Data Type Conversion6/1 -> Bus Creator/5
  Data Type Conversion5/1 -> Bus Creator/4
  Data Type Conversion7/1 -> Bus Creator/3
  Data Type Conversion8/1 -> Bus Creator/2
  Data Type Conversion4/1 -> Bus Creator/1

== system controller_dev_sg_HIL_noTP/UDP to Mapping and Localization (Position, IMU, Wheelspeed)5 ==
  VehicleSensorData : Inport
  Enable : EnablePort
  Bus Creator : BusCreator  Inputs=12
  Bus Selector : BusSelector  OutputSignals=x_Loc1_m,y_Loc1_m,psi_YawAngleLoc1_rad,vx_CoGVel1_mps,vy_CoGVel1_mps,dPsi_YawRateIMU1_radps,ax_CoGIMU1_mps2,ay_CoGIMU1_mps2,omega_WheelFL_radps,omega_WheelFR_radps,omega_WheelRL_radps,omega_WheelRR_radps
  Byte Packing 3 : xpcutilitieslib/Byte Packing   MaskPackedDataType=uint8  MaskUnpackedDataTypes={'double'}  MaskAlignment=1
  Data Type Conversion{,1..8,12..14} (12 alike) : DataTypeConversion  OutDataTypeStr=double
  UDP Send1 : xpcrtudplib/UDP Send  ipAddressVal=10.0.0.20  localPort=40563  toAddress=10.0.0.16  toPort=ModMapLoc_VehSenDat_SendPort  sampleTime=-1
      settings: SourceProductName=Simulink Real-Time  SourceProductBaseCode=XP
  Width : Width
  wires:
  VehicleSensorData/1 -> Bus Selector/1
  Byte Packing 3/1 -> Width/1, UDP Send1/1
  Width/1 -> UDP Send1/2
  Bus Creator/1 -> Byte Packing 3/1
  Bus Selector/12 -> Data Type Conversion13/1  "<omega_WheelRR_radps>"
  Bus Selector/11 -> Data Type Conversion12/1  "<omega_WheelRL_radps>"
  Bus Selector/10 -> Data Type Conversion14/1  "<omega_WheelFR_radps>"
  Bus Selector/9 -> Data Type Conversion1/1  "<omega_WheelFL_radps>"
  Bus Selector/7 -> Data Type Conversion3/1  "<ax_CoGIMU1_mps2>"
  Bus Selector/8 -> Data Type Conversion2/1  "<ay_CoGIMU1_mps2>"
  Bus Selector/6 -> Data Type Conversion/1  "<dPsi_YawRateIMU1_radps>"
  Bus Selector/1 -> Data Type Conversion4/1  "<x_Loc1_m>"
  Bus Selector/2 -> Data Type Conversion8/1  "<y_Loc1_m>"
  Bus Selector/3 -> Data Type Conversion7/1  "<psi_YawAngleLoc1_rad>"
  Bus Selector/4 -> Data Type Conversion5/1  "<vx_CoGVel1_mps>"
  Bus Selector/5 -> Data Type Conversion6/1  "<vy_CoGVel1_mps>"
  Data Type Conversion12/1 -> Bus Creator/11
  Data Type Conversion13/1 -> Bus Creator/12
  Data Type Conversion14/1 -> Bus Creator/10
  Data Type Conversion1/1 -> Bus Creator/9
  Data Type Conversion3/1 -> Bus Creator/7
  Data Type Conversion2/1 -> Bus Creator/8
  Data Type Conversion/1 -> Bus Creator/6
  Data Type Conversion6/1 -> Bus Creator/5
  Data Type Conversion5/1 -> Bus Creator/4
  Data Type Conversion7/1 -> Bus Creator/3
  Data Type Conversion8/1 -> Bus Creator/2
  Data Type Conversion4/1 -> Bus Creator/1

== system controller_dev_sg_HIL_noTP/UDP to Mapping and Localization (Position, IMU, Wheelspeed)6 ==
  VehicleSensorData : Inport
  Enable : EnablePort
  Bus Creator : BusCreator  Inputs=12
  Bus Selector : BusSelector  OutputSignals=x_Loc1_m,y_Loc1_m,psi_YawAngleLoc1_rad,vx_CoGVel1_mps,vy_CoGVel1_mps,dPsi_YawRateIMU1_radps,ax_CoGIMU1_mps2,ay_CoGIMU1_mps2,omega_WheelFL_radps,omega_WheelFR_radps,omega_WheelRL_radps,omega_WheelRR_radps
  Byte Packing 3 : xpcutilitieslib/Byte Packing   MaskPackedDataType=uint8  MaskUnpackedDataTypes={'double'}  MaskAlignment=1
  Data Type Conversion{,1..8,12..14} (12 alike) : DataTypeConversion  OutDataTypeStr=double
  UDP Send1 : xpcrtudplib/UDP Send  ipAddressVal=10.0.0.20  localPort=40573  toAddress=10.0.0.17  toPort=ModMapLoc_VehSenDat_SendPort  sampleTime=-1
      settings: SourceProductName=Simulink Real-Time  SourceProductBaseCode=XP
  Width : Width
  wires:
  VehicleSensorData/1 -> Bus Selector/1
  Byte Packing 3/1 -> Width/1, UDP Send1/1
  Width/1 -> UDP Send1/2
  Bus Creator/1 -> Byte Packing 3/1
  Bus Selector/12 -> Data Type Conversion13/1  "<omega_WheelRR_radps>"
  Bus Selector/11 -> Data Type Conversion12/1  "<omega_WheelRL_radps>"
  Bus Selector/10 -> Data Type Conversion14/1  "<omega_WheelFR_radps>"
  Bus Selector/9 -> Data Type Conversion1/1  "<omega_WheelFL_radps>"
  Bus Selector/7 -> Data Type Conversion3/1  "<ax_CoGIMU1_mps2>"
  Bus Selector/8 -> Data Type Conversion2/1  "<ay_CoGIMU1_mps2>"
  Bus Selector/6 -> Data Type Conversion/1  "<dPsi_YawRateIMU1_radps>"
  Bus Selector/1 -> Data Type Conversion4/1  "<x_Loc1_m>"
  Bus Selector/2 -> Data Type Conversion8/1  "<y_Loc1_m>"
  Bus Selector/3 -> Data Type Conversion7/1  "<psi_YawAngleLoc1_rad>"
  Bus Selector/4 -> Data Type Conversion5/1  "<vx_CoGVel1_mps>"
  Bus Selector/5 -> Data Type Conversion6/1  "<vy_CoGVel1_mps>"
  Data Type Conversion12/1 -> Bus Creator/11
  Data Type Conversion13/1 -> Bus Creator/12
  Data Type Conversion14/1 -> Bus Creator/10
  Data Type Conversion1/1 -> Bus Creator/9
  Data Type Conversion3/1 -> Bus Creator/7
  Data Type Conversion2/1 -> Bus Creator/8
  Data Type Conversion/1 -> Bus Creator/6
  Data Type Conversion6/1 -> Bus Creator/5
  Data Type Conversion5/1 -> Bus Creator/4
  Data Type Conversion7/1 -> Bus Creator/3
  Data Type Conversion8/1 -> Bus Creator/2
  Data Type Conversion4/1 -> Bus Creator/1

== system controller_dev_sg_HIL_noTP/UDP to Mapping and Localization (Position, IMU, Wheelspeed)7 ==
  VehicleSensorData : Inport
  Enable : EnablePort
  Bus Creator : BusCreator  Inputs=12
  Bus Selector : BusSelector  OutputSignals=x_Loc1_m,y_Loc1_m,psi_YawAngleLoc1_rad,vx_CoGVel1_mps,vy_CoGVel1_mps,dPsi_YawRateIMU1_radps,ax_CoGIMU1_mps2,ay_CoGIMU1_mps2,omega_WheelFL_radps,omega_WheelFR_radps,omega_WheelRL_radps,omega_WheelRR_radps
  Byte Packing 3 : xpcutilitieslib/Byte Packing   MaskPackedDataType=uint8  MaskUnpackedDataTypes={'double'}  MaskAlignment=1
  Data Type Conversion{,1..8,12..14} (12 alike) : DataTypeConversion  OutDataTypeStr=double
  UDP Send1 : xpcrtudplib/UDP Send  ipAddressVal=10.0.0.20  localPort=40583  toAddress=10.0.0.18  toPort=ModMapLoc_VehSenDat_SendPort  sampleTime=-1
      settings: SourceProductName=Simulink Real-Time  SourceProductBaseCode=XP
  Width : Width
  wires:
  VehicleSensorData/1 -> Bus Selector/1
  Byte Packing 3/1 -> Width/1, UDP Send1/1
  Width/1 -> UDP Send1/2
  Bus Creator/1 -> Byte Packing 3/1
  Bus Selector/12 -> Data Type Conversion13/1  "<omega_WheelRR_radps>"
  Bus Selector/11 -> Data Type Conversion12/1  "<omega_WheelRL_radps>"
  Bus Selector/10 -> Data Type Conversion14/1  "<omega_WheelFR_radps>"
  Bus Selector/9 -> Data Type Conversion1/1  "<omega_WheelFL_radps>"
  Bus Selector/7 -> Data Type Conversion3/1  "<ax_CoGIMU1_mps2>"
  Bus Selector/8 -> Data Type Conversion2/1  "<ay_CoGIMU1_mps2>"
  Bus Selector/6 -> Data Type Conversion/1  "<dPsi_YawRateIMU1_radps>"
  Bus Selector/1 -> Data Type Conversion4/1  "<x_Loc1_m>"
  Bus Selector/2 -> Data Type Conversion8/1  "<y_Loc1_m>"
  Bus Selector/3 -> Data Type Conversion7/1  "<psi_YawAngleLoc1_rad>"
  Bus Selector/4 -> Data Type Conversion5/1  "<vx_CoGVel1_mps>"
  Bus Selector/5 -> Data Type Conversion6/1  "<vy_CoGVel1_mps>"
  Data Type Conversion12/1 -> Bus Creator/11
  Data Type Conversion13/1 -> Bus Creator/12
  Data Type Conversion14/1 -> Bus Creator/10
  Data Type Conversion1/1 -> Bus Creator/9
  Data Type Conversion3/1 -> Bus Creator/7
  Data Type Conversion2/1 -> Bus Creator/8
  Data Type Conversion/1 -> Bus Creator/6
  Data Type Conversion6/1 -> Bus Creator/5
  Data Type Conversion5/1 -> Bus Creator/4
  Data Type Conversion7/1 -> Bus Creator/3
  Data Type Conversion8/1 -> Bus Creator/2
  Data Type Conversion4/1 -> Bus Creator/1
